simulink model "LockInResistanceMeasurementMethod"  (R2020b)
settings: Solver=VariableStepAuto  StartTime=0.0  StopTime=0.25  RelTol=1e-3
libraries: powerlib x11, powerlib_meascontrol x5
settings Model: Creator=Yang Ting  LastModifiedBy=Photonics_Lab

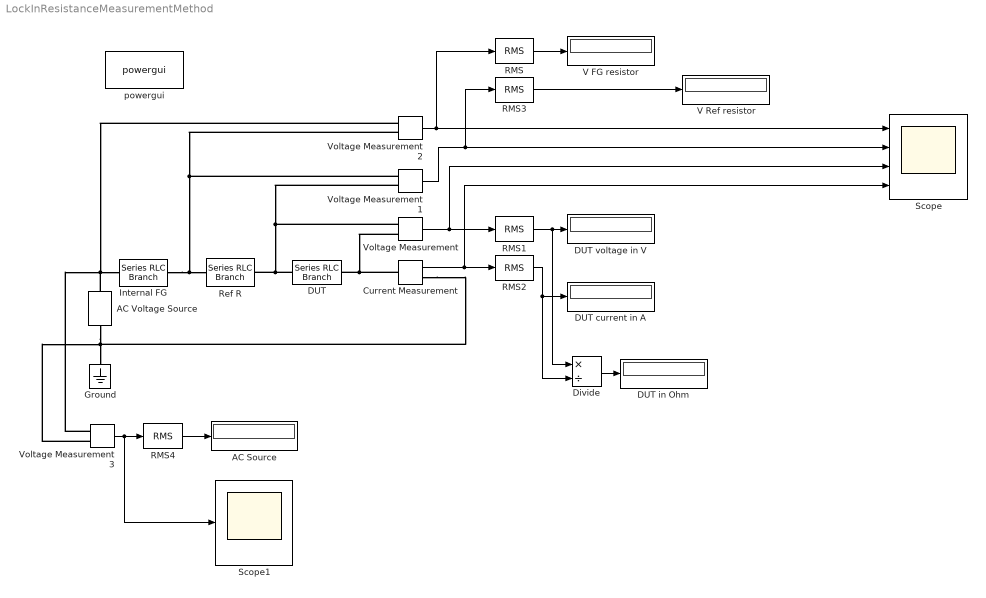
== system LockInResistanceMeasurementMethod ==
  AC Source : Display
  AC Voltage Source : powerlib/Electrical Sources/AC Voltage Source  Amplitude=0.53  Phase=0  Frequency=5  SampleTime=0  Measurements=None  BusType=swing  Pref=10e3  Qref=0  Qmin=-inf  Qmax=+inf
  Current Measurement : powerlib/Measurements/Current Measurement  PhasorSimulation=off  OutputType=Complex  PSBequivalent=0
  DUT : powerlib/Elements/Series RLC Branch  LConnTagsString=__new0  RConnTagsString=__new0  BranchType=R  Resistance=81  Inductance=1e-3  SetiL0=off  InitialCurrent=0  Capacitance=1e-6  Setx0=off  InitialVoltage=0  Measurements=None
  DUT current in A : Display
  DUT in Ohm : Display
  DUT voltage in V : Display
  Divide : Product  Inputs=*/
  Ground : powerlib/Elements/Ground  LConnTagsString=a
  Internal FG : powerlib/Elements/Series RLC Branch  Tag=Internal  LConnTagsString=__new0  RConnTagsString=__new0  BranchType=R  Resistance=50  Inductance=1e-3  SetiL0=off  InitialCurrent=0  Capacitance=1e-6  Setx0=off  InitialVoltage=0  Measurements=None
  RMS{,1..4} (5 alike) : powerlib_meascontrol/Measurements/RMS  TrueRMS=on  Freq=10  RMSInit=0  Ts=0
  Ref R : powerlib/Elements/Series RLC Branch  LConnTagsString=__new0  RConnTagsString=__new0  BranchType=R  Resistance=124e3  Inductance=1e-3  SetiL0=off  InitialCurrent=0  Capacitance=1e-6  Setx0=off  InitialVoltage=0  Measurements=None
  Scope : Scope  NumInputPorts=4
  Scope1 : Scope
  V FG resistor : Display
  V Ref resistor : Display
  Voltage Measurement{,1..3} (4 alike) : powerlib/Measurements/Voltage Measurement  PhasorSimulation=off  OutputType=Complex  PSBequivalent=0
  powergui : powerlib/powergui  Priority=1  SimulationMode=Continuous  SampleTime=50e-6  frequency=60  Iterations=50  frequencyindice=5  Pbase=100e6  ErrMax=1e-4  UnitsV=kV  UnitsW=MW  buscounter=0  FunctionMessages=off  echomessages=off  EnableUseOfTLC=off  CurrentSourceSwitches=off  DisableSnubberDevices=off  DisableRonSwitches=off  DisableVfSwitches=off  DisplayEquations=off  AutomaticDiscreteSolvers=off  SolverType=Tustin/Backward Euler (TBE)  Interpol=off  ExternalGateDelay=off  methode=off  Ts=100  x0status=blocks  SPID=on  SwTol=0  HookPort=off  NonlinearTolerance=1e-4  nMaxIteration=100  ContinueOnMaxIteration=off  RestoreLinks=warning  ResistiveCurrentMeasurement=off  Frange=[0:2:500]  Ylog=off  Xlog=on  ShowGrid=off  save=off  variable=ZData  structure=0  ZoomFFT=off  StartTime=0.0  cycles=1  DisplayStyle=1  fundamental=60  FreqAxis=off  MaxFrequency=1000  frequencyindicesteady=1  RmsSteady=1  display=off
  wires:
  Voltage Measurement2/1 -> RMS/1, Scope/1
  Voltage Measurement1/1 -> RMS3/1, Scope/2
  Voltage Measurement/1 -> RMS1/1, Scope/3
  Current Measurement/1 -> Scope/4, RMS2/1
  RMS/1 -> V FG resistor/1
  RMS1/1 -> Divide/1, DUT voltage in V/1
  RMS2/1 -> Divide/2, DUT current in A/1
  RMS3/1 -> V Ref resistor/1
  Divide/1 -> DUT in Ohm/1
  Voltage Measurement3/1 -> Scope1/1, RMS4/1
  RMS4/1 -> AC Source/1
  connections:
  AC Voltage Source/RConn1 -- Voltage Measurement3/LConn1 -- Internal FG/LConn1 -- Voltage Measurement2/LConn1
  AC Voltage Source/LConn1 -- Voltage Measurement3/LConn2 -- Ground/LConn1 -- Current Measurement/RConn1
  DUT/LConn1 -- Voltage Measurement1/LConn2 -- Voltage Measurement/LConn1 -- Ref R/RConn1
  Internal FG/RConn1 -- Voltage Measurement2/LConn2 -- Voltage Measurement1/LConn1 -- Ref R/LConn1
  Voltage Measurement/LConn2 -- Current Measurement/LConn1 -- DUT/RConn1
